simulink model "Regressao9_6"  (R2012b)
settings: Solver=FixedStepDiscrete  SolverMode=SingleTasking  StartTime=0.0  StopTime=limSim  FixedStep=ts  RelTol=1e-3
libraries: xbsIndex_r4 x399, roblocks x1
settings Model: Creator=snata  LastModifiedBy=snata

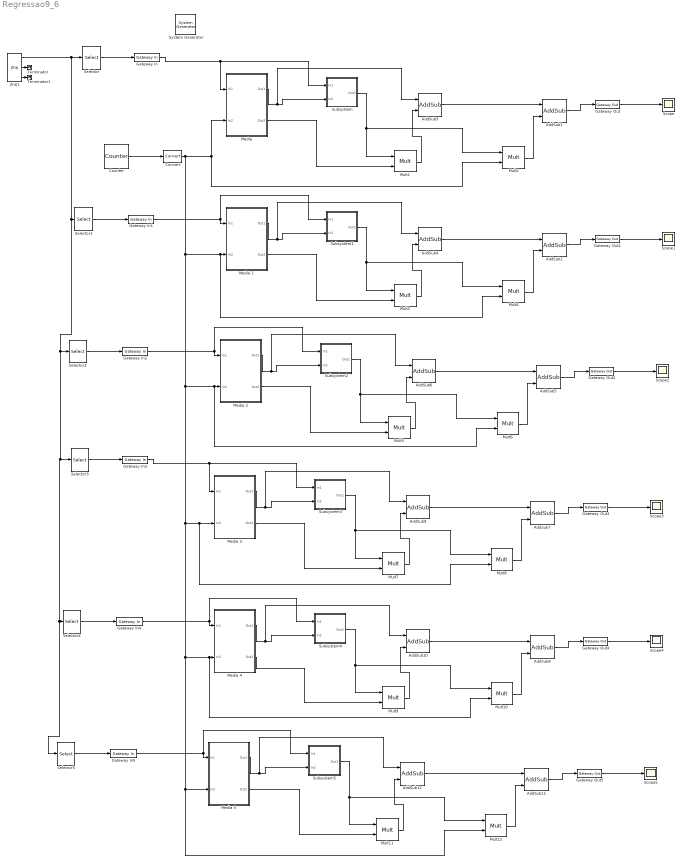
== system Regressao9_6 ==
  " System Generator" : xbsIndex_r4/ System Generator  Tag=genX  xilinxfamily=virtex6  part=xc6vlx240t  speed=-1  package=ff1156  synthesis_tool=XST  clock_wrapper=Clock Enables  directory=C:/Users/snata/Documents/Linear_Predictors/Regressao9/netlist6  proj_type=Project Navigator  Synth_file=XST Defaults  Impl_file=ISE Defaults  testbench=off  simulink_period=ts  sysclk_period=10  dcm_input_clock_period=10  incr_netlist=off  trim_vbits=Everywhere in SubSystem  dbl_ovrd=According to Block Masks  core_generation=According to Block Masks  run_coregen=off  deprecated_control=off  eval_field=0  block_type=sysgen
  AddSub{1..2,5,7..8,11} (6 alike) : xbsIndex_r4/AddSub  mode=Addition  use_carryin=off  use_carryout=off  en=off  latency=0  precision=Full  arith_type=Unsigned  n_bits=16  bin_pt=14  quantization=Truncate  overflow=Wrap  dbl_ovrd=off  use_behavioral_HDL=off  hw_selection=Fabric  pipelined=off  block_type=addsub
  AddSub{3..4,6,9..10,12} (6 alike) : xbsIndex_r4/AddSub  mode=Subtraction  use_carryin=off  use_carryout=off  en=off  latency=0  precision=Full  arith_type=Unsigned  n_bits=16  bin_pt=14  quantization=Truncate  overflow=Wrap  dbl_ovrd=off  use_behavioral_HDL=off  hw_selection=Fabric  pipelined=off  block_type=addsub
  Convert : xbsIndex_r4/Convert  gui_display_data_type=Floating-point  arith_type=Floating-point  n_bits=16  bin_pt=14  float_type=Single  exp_bits=8  fraction_bits=24  quantization=Truncate  overflow=Wrap  en=off  latency=0  dbl_ovrd=off  pipeline=off  block_type=convert
  Counter : xbsIndex_r4/Counter  cnt_type=Free Running  cnt_to=Inf  operation=Up  start_count=0  cnt_by_val=1  arith_type="Signed  (2's comp)"  n_bits=32  bin_pt=1  load_pin=off  rst=off  en=off  explicit_period=on  period=ts  dbl_ovrd=off  use_behavioral_HDL=off  implementation=Fabric  block_type=counter
  Gateway In{,1..5} (6 alike) : xbsIndex_r4/Gateway In  gui_display_data_type=Floating-point  arith_type=Floating-point  n_bits=16  bin_pt=14  preci_type=Single  exp_width=8  frac_width=24  quantization="Round  (unbiased: +/- Inf)"  overflow=Saturate  period=ts  dbl_ovrd=off  timing_constraint=None  locs_specified=off  LOCs={}  UseAsADC=off  ADCChannel='1'  inherit_from_input=off  hdl_port=on  block_type=gatewayin
  Gateway Out{,1..5} (6 alike) : xbsIndex_r4/Gateway Out  inherit_from_input=off  hdl_port=on  timing_constraint=None  locs_specified=off  LOCs={}  UseAsDAC=off  DACChannel='1'  block_type=gatewayout
  "Media " : Subsystem
  Media 1 : Subsystem
  Media 2 : Subsystem
  Media 3 : Subsystem
  Media 4 : Subsystem
  Media 5 : Subsystem
  Mult{1..12} (12 alike) : xbsIndex_r4/Mult  precision=Full  arith_type="Signed  (2's comp)"  n_bits=16  bin_pt=14  quantization=Truncate  overflow=Wrap  en=off  latency=0  dbl_ovrd=off  use_behavioral_HDL=off  opt=Speed  use_embedded=on  optimum_pipeline=off  pipeline=on  use_rpm=on  placement_style=Triangular  block_type=mult
  Scope{,1..5} (6 alike) : Scope
      Scope settings: YMin=5.55112e-17  YMax=1.6
      Scope1 settings: YMin=5.55112e-17  YMax=1.6
      Scope2 settings: YMin=5.55112e-17  YMax=1.6  SaveName=ScopeData2
      Scope3 settings: YMin=5.55112e-17  YMax=1.6  SaveName=ScopeData3
      Scope4 settings: YMin=5.55112e-17  YMax=1.6  SaveName=ScopeData4
      Scope5 settings: YMin=5.55112e-17  YMax=1.6  SaveName=ScopeData5
  Selector{,1..5} (6 alike) : Selector  InputPortWidth=3  IndexOptions=Index vector (dialog)  Indices=[1]  OutputSizes=1
  Subsystem : Subsystem
  Subsystem1 : Subsystem
  Subsystem2 : Subsystem
  Subsystem3 : Subsystem
  Subsystem4 : Subsystem
  Subsystem5 : Subsystem
  Terminator : Terminator
  Terminator1 : Terminator
  jtraj1 : roblocks/Trajectory/jtraj  q0=[0 -pi/2 pi]  qf=[pi/2 pi/4 pi/2]  tmax=limSim  ts=ts
  wires:
  Selector/1 -> Gateway In/1
  Gateway In/1 -> Subsystem/1(In1), "Media "/1(In1)
  AddSub1/1 -> Gateway Out/1
  Gateway Out/1 -> Scope/1
  "Media "/1(Out1) -> AddSub3/1, Subsystem/2(In2)
  Counter/1 -> Convert/1
  Mult1/1 -> AddSub3/2
  AddSub3/1 -> AddSub1/1
  Mult2/1 -> AddSub1/2
  Subsystem/1(Out1) -> Mult2/1, Mult1/1
  "Media "/2(Out2) -> Mult1/2
  Selector1/1 -> Gateway In1/1
  Gateway In1/1 -> Subsystem1/1(In1), Media 1/1(In1)
  AddSub2/1 -> Gateway Out1/1
  Gateway Out1/1 -> Scope1/1
  Media 1/1(Out1) -> AddSub4/1, Subsystem1/2(In2)
  Mult3/1 -> AddSub4/2
  AddSub4/1 -> AddSub2/1
  Mult4/1 -> AddSub2/2
  Subsystem1/1(Out1) -> Mult4/1, Mult3/1
  Media 1/2(Out2) -> Mult3/2
  Selector2/1 -> Gateway In2/1
  Gateway In2/1 -> Subsystem2/1(In1), Media 2/1(In1)
  AddSub5/1 -> Gateway Out2/1
  Gateway Out2/1 -> Scope2/1
  Media 2/1(Out1) -> AddSub6/1, Subsystem2/2(In2)
  Mult5/1 -> AddSub6/2
  AddSub6/1 -> AddSub5/1
  Mult6/1 -> AddSub5/2
  Subsystem2/1(Out1) -> Mult6/1, Mult5/1
  Media 2/2(Out2) -> Mult5/2
  Selector3/1 -> Gateway In3/1
  Gateway In3/1 -> Subsystem3/1(In1), Media 3/1(In1)
  AddSub7/1 -> Gateway Out3/1
  Gateway Out3/1 -> Scope3/1
  Media 3/1(Out1) -> AddSub9/1, Subsystem3/2(In2)
  Mult7/1 -> AddSub9/2
  AddSub9/1 -> AddSub7/1
  Mult8/1 -> AddSub7/2
  Subsystem3/1(Out1) -> Mult8/1, Mult7/1
  Media 3/2(Out2) -> Mult7/2
  Selector4/1 -> Gateway In4/1
  jtraj1/1 -> Selector5/1, Selector4/1, Selector3/1, Selector2/1, Selector1/1, Selector/1
  Gateway In4/1 -> Subsystem4/1(In1), Media 4/1(In1)
  AddSub8/1 -> Gateway Out4/1
  Gateway Out4/1 -> Scope4/1
  Media 4/1(Out1) -> AddSub10/1, Subsystem4/2(In2)
  Mult9/1 -> AddSub10/2
  AddSub10/1 -> AddSub8/1
  Mult10/1 -> AddSub8/2
  Subsystem4/1(Out1) -> Mult10/1, Mult9/1
  Media 4/2(Out2) -> Mult9/2
  Selector5/1 -> Gateway In5/1
  Gateway In5/1 -> Subsystem5/1(In1), Media 5/1(In1)
  AddSub11/1 -> Gateway Out5/1
  Gateway Out5/1 -> Scope5/1
  Media 5/1(Out1) -> AddSub12/1, Subsystem5/2(In2)
  Convert/1 -> Mult4/2, Media 1/2(In2), Mult6/2, Media 2/2(In2), Mult8/2, Media 3/2(In2), Mult10/2, Media 4/2(In2), Media 5/2(In2), Mult12/2, "Media "/2(In2), Mult2/2
  Mult11/1 -> AddSub12/2
  AddSub12/1 -> AddSub11/1
  Mult12/1 -> AddSub11/2
  Subsystem5/1(Out1) -> Mult12/1, Mult11/1
  Media 5/2(Out2) -> Mult11/2
  jtraj1/2 -> Terminator/1
  jtraj1/3 -> Terminator1/1

== system Regressao9_6/Media  ==
  In1 : Inport
  In2 : Inport  Port=2
  CMult : xbsIndex_r4/CMult  const=1/10  gui_display_data_type=Floating-point  const_n_bits=16  const_bin_pt=14  float_type=Single  exp_bits=8  fraction_bits=24  en=off  latency=0  precision=Full  arith_type="Signed  (2's comp)"  n_bits=16  bin_pt=14  quantization=Truncate  overflow=Wrap  dbl_ovrd=off  use_behavioral_HDL=off  mem_type=Distributed RAM  pipeline=off  block_type=cmult
  CMult1 : xbsIndex_r4/CMult  const=1/10  gui_display_data_type=Floating-point  const_n_bits=16  const_bin_pt=14  float_type=Single  exp_bits=8  fraction_bits=24  en=off  latency=0  precision=Full  arith_type="Signed  (2's comp)"  n_bits=16  bin_pt=14  quantization=Truncate  overflow=Wrap  dbl_ovrd=off  use_behavioral_HDL=off  mem_type=Distributed RAM  pipeline=off  block_type=cmult
  Soma : Subsystem
  Soma1 : Subsystem
  Out1 : Outport
  Out2 : Outport  Port=2
  wires:
  In1/1 -> Soma/1(In1)
  Soma/1(Out1) -> CMult/1
  CMult/1 -> Out1/1
  In2/1 -> Soma1/1(In1)
  Soma1/1(Out1) -> CMult1/1
  CMult1/1 -> Out2/1

== system Regressao9_6/Media 1 ==
  In1 : Inport
  In2 : Inport  Port=2
  CMult : xbsIndex_r4/CMult  const=1/10  gui_display_data_type=Floating-point  const_n_bits=16  const_bin_pt=14  float_type=Single  exp_bits=8  fraction_bits=24  en=off  latency=0  precision=Full  arith_type="Signed  (2's comp)"  n_bits=16  bin_pt=14  quantization=Truncate  overflow=Wrap  dbl_ovrd=off  use_behavioral_HDL=off  mem_type=Distributed RAM  pipeline=off  block_type=cmult
  CMult1 : xbsIndex_r4/CMult  const=1/10  gui_display_data_type=Floating-point  const_n_bits=16  const_bin_pt=14  float_type=Single  exp_bits=8  fraction_bits=24  en=off  latency=0  precision=Full  arith_type="Signed  (2's comp)"  n_bits=16  bin_pt=14  quantization=Truncate  overflow=Wrap  dbl_ovrd=off  use_behavioral_HDL=off  mem_type=Distributed RAM  pipeline=off  block_type=cmult
  Soma : Subsystem
  Soma1 : Subsystem
  Out1 : Outport
  Out2 : Outport  Port=2
  wires:
  In1/1 -> Soma/1(In1)
  Soma/1(Out1) -> CMult/1
  CMult/1 -> Out1/1
  In2/1 -> Soma1/1(In1)
  Soma1/1(Out1) -> CMult1/1
  CMult1/1 -> Out2/1

== system Regressao9_6/Media 2 ==
  In1 : Inport
  In2 : Inport  Port=2
  CMult : xbsIndex_r4/CMult  const=1/10  gui_display_data_type=Floating-point  const_n_bits=16  const_bin_pt=14  float_type=Single  exp_bits=8  fraction_bits=24  en=off  latency=0  precision=Full  arith_type="Signed  (2's comp)"  n_bits=16  bin_pt=14  quantization=Truncate  overflow=Wrap  dbl_ovrd=off  use_behavioral_HDL=off  mem_type=Distributed RAM  pipeline=off  block_type=cmult
  CMult1 : xbsIndex_r4/CMult  const=1/10  gui_display_data_type=Floating-point  const_n_bits=16  const_bin_pt=14  float_type=Single  exp_bits=8  fraction_bits=24  en=off  latency=0  precision=Full  arith_type="Signed  (2's comp)"  n_bits=16  bin_pt=14  quantization=Truncate  overflow=Wrap  dbl_ovrd=off  use_behavioral_HDL=off  mem_type=Distributed RAM  pipeline=off  block_type=cmult
  Soma : Subsystem
  Soma1 : Subsystem
  Out1 : Outport
  Out2 : Outport  Port=2
  wires:
  In1/1 -> Soma/1(In1)
  Soma/1(Out1) -> CMult/1
  CMult/1 -> Out1/1
  In2/1 -> Soma1/1(In1)
  Soma1/1(Out1) -> CMult1/1
  CMult1/1 -> Out2/1

== system Regressao9_6/Media 3 ==
  In1 : Inport
  In2 : Inport  Port=2
  CMult : xbsIndex_r4/CMult  const=1/10  gui_display_data_type=Floating-point  const_n_bits=16  const_bin_pt=14  float_type=Single  exp_bits=8  fraction_bits=24  en=off  latency=0  precision=Full  arith_type="Signed  (2's comp)"  n_bits=16  bin_pt=14  quantization=Truncate  overflow=Wrap  dbl_ovrd=off  use_behavioral_HDL=off  mem_type=Distributed RAM  pipeline=off  block_type=cmult
  CMult1 : xbsIndex_r4/CMult  const=1/10  gui_display_data_type=Floating-point  const_n_bits=16  const_bin_pt=14  float_type=Single  exp_bits=8  fraction_bits=24  en=off  latency=0  precision=Full  arith_type="Signed  (2's comp)"  n_bits=16  bin_pt=14  quantization=Truncate  overflow=Wrap  dbl_ovrd=off  use_behavioral_HDL=off  mem_type=Distributed RAM  pipeline=off  block_type=cmult
  Soma : Subsystem
  Soma1 : Subsystem
  Out1 : Outport
  Out2 : Outport  Port=2
  wires:
  In1/1 -> Soma/1(In1)
  Soma/1(Out1) -> CMult/1
  CMult/1 -> Out1/1
  In2/1 -> Soma1/1(In1)
  Soma1/1(Out1) -> CMult1/1
  CMult1/1 -> Out2/1

== system Regressao9_6/Media 4 ==
  In1 : Inport
  In2 : Inport  Port=2
  CMult : xbsIndex_r4/CMult  const=1/10  gui_display_data_type=Floating-point  const_n_bits=16  const_bin_pt=14  float_type=Single  exp_bits=8  fraction_bits=24  en=off  latency=0  precision=Full  arith_type="Signed  (2's comp)"  n_bits=16  bin_pt=14  quantization=Truncate  overflow=Wrap  dbl_ovrd=off  use_behavioral_HDL=off  mem_type=Distributed RAM  pipeline=off  block_type=cmult
  CMult1 : xbsIndex_r4/CMult  const=1/10  gui_display_data_type=Floating-point  const_n_bits=16  const_bin_pt=14  float_type=Single  exp_bits=8  fraction_bits=24  en=off  latency=0  precision=Full  arith_type="Signed  (2's comp)"  n_bits=16  bin_pt=14  quantization=Truncate  overflow=Wrap  dbl_ovrd=off  use_behavioral_HDL=off  mem_type=Distributed RAM  pipeline=off  block_type=cmult
  Soma : Subsystem
  Soma1 : Subsystem
  Out1 : Outport
  Out2 : Outport  Port=2
  wires:
  In1/1 -> Soma/1(In1)
  Soma/1(Out1) -> CMult/1
  CMult/1 -> Out1/1
  In2/1 -> Soma1/1(In1)
  Soma1/1(Out1) -> CMult1/1
  CMult1/1 -> Out2/1

== system Regressao9_6/Media 5 ==
  In1 : Inport
  In2 : Inport  Port=2
  CMult : xbsIndex_r4/CMult  const=1/10  gui_display_data_type=Floating-point  const_n_bits=16  const_bin_pt=14  float_type=Single  exp_bits=8  fraction_bits=24  en=off  latency=0  precision=Full  arith_type="Signed  (2's comp)"  n_bits=16  bin_pt=14  quantization=Truncate  overflow=Wrap  dbl_ovrd=off  use_behavioral_HDL=off  mem_type=Distributed RAM  pipeline=off  block_type=cmult
  CMult1 : xbsIndex_r4/CMult  const=1/10  gui_display_data_type=Floating-point  const_n_bits=16  const_bin_pt=14  float_type=Single  exp_bits=8  fraction_bits=24  en=off  latency=0  precision=Full  arith_type="Signed  (2's comp)"  n_bits=16  bin_pt=14  quantization=Truncate  overflow=Wrap  dbl_ovrd=off  use_behavioral_HDL=off  mem_type=Distributed RAM  pipeline=off  block_type=cmult
  Soma : Subsystem
  Soma1 : Subsystem
  Out1 : Outport
  Out2 : Outport  Port=2
  wires:
  In1/1 -> Soma/1(In1)
  Soma/1(Out1) -> CMult/1
  CMult/1 -> Out1/1
  In2/1 -> Soma1/1(In1)
  Soma1/1(Out1) -> CMult1/1
  CMult1/1 -> Out2/1

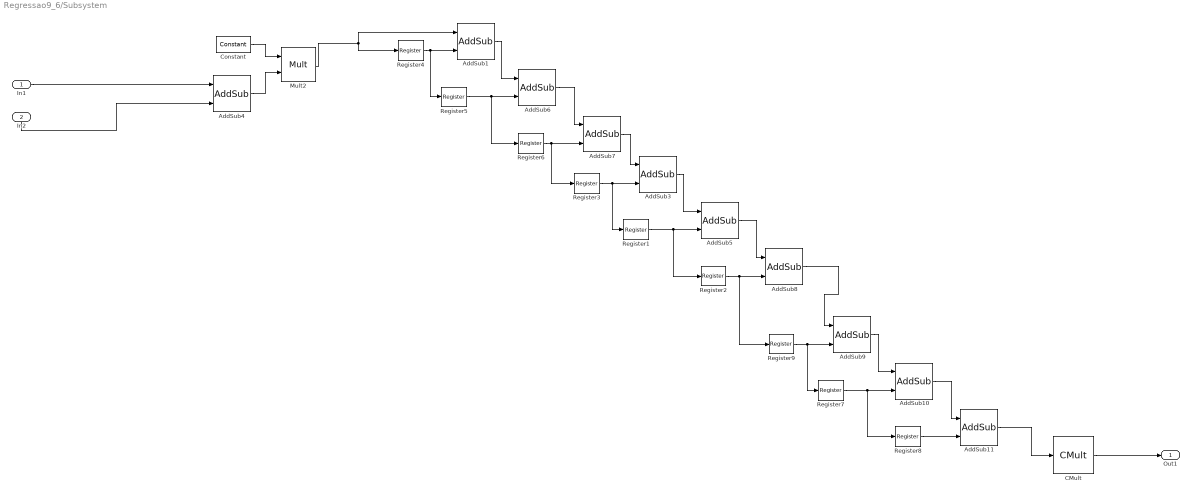
== system Regressao9_6/Subsystem ==
  In1 : Inport
  In2 : Inport  Port=2
  AddSub{1,3,5..11} (9 alike) : xbsIndex_r4/AddSub  mode=Addition  use_carryin=off  use_carryout=off  en=off  latency=0  precision=Full  arith_type=Unsigned  n_bits=16  bin_pt=14  quantization=Truncate  overflow=Wrap  dbl_ovrd=off  use_behavioral_HDL=off  hw_selection=Fabric  pipelined=off  block_type=addsub
  AddSub4 : xbsIndex_r4/AddSub  mode=Subtraction  use_carryin=off  use_carryout=off  en=off  latency=0  precision=Full  arith_type=Unsigned  n_bits=16  bin_pt=14  quantization=Truncate  overflow=Wrap  dbl_ovrd=off  use_behavioral_HDL=off  hw_selection=Fabric  pipelined=off  block_type=addsub
  CMult : xbsIndex_r4/CMult  const=1/20.25  gui_display_data_type=Floating-point  const_n_bits=16  const_bin_pt=14  float_type=Single  exp_bits=8  fraction_bits=24  en=off  latency=0  precision=Full  arith_type="Signed  (2's comp)"  n_bits=16  bin_pt=14  quantization=Truncate  overflow=Wrap  dbl_ovrd=off  use_behavioral_HDL=off  mem_type=Distributed RAM  pipeline=off  block_type=cmult
  Constant : xbsIndex_r4/Constant  const=4.5  gui_display_data_type=Floating-point  arith_type=Floating-point  n_bits=16  bin_pt=14  preci_type=Single  exp_width=8  frac_width=24  explicit_period=off  period=1  equ=P=C  opselect=C  inp2=PCIN>>17  opr=+  inp1=P  carry=CIN  dbl_ovrd=off  block_type=constant
  Mult2 : xbsIndex_r4/Mult  precision=Full  arith_type="Signed  (2's comp)"  n_bits=16  bin_pt=14  quantization=Truncate  overflow=Wrap  en=off  latency=0  dbl_ovrd=off  use_behavioral_HDL=off  opt=Speed  use_embedded=on  optimum_pipeline=off  pipeline=on  use_rpm=on  placement_style=Triangular  block_type=mult
  Register{1..9} (9 alike) : xbsIndex_r4/Register  init=0  rst=off  en=off  dbl_ovrd=off  block_type=register
  Out1 : Outport
  wires:
  CMult/1 -> Out1/1
  AddSub4/1 -> Mult2/2
  In1/1 -> AddSub4/1
  In2/1 -> AddSub4/2
  AddSub11/1 -> CMult/1
  Mult2/1 -> Register4/1, AddSub1/1
  AddSub6/1 -> AddSub7/1
  AddSub1/1 -> AddSub6/1
  Register4/1 -> Register5/1, AddSub1/2
  Register5/1 -> Register6/1, AddSub6/2
  Register6/1 -> Register3/1, AddSub7/2
  AddSub5/1 -> AddSub8/1
  AddSub3/1 -> AddSub5/1
  Register3/1 -> Register1/1, AddSub3/2
  Register1/1 -> Register2/1, AddSub5/2
  AddSub7/1 -> AddSub3/1
  Register2/1 -> Register9/1, AddSub8/2
  AddSub10/1 -> AddSub11/1
  AddSub9/1 -> AddSub10/1
  Register9/1 -> AddSub9/2, Register7/1
  Register7/1 -> AddSub10/2, Register8/1
  Register8/1 -> AddSub11/2
  AddSub8/1 -> AddSub9/1
  Constant/1 -> Mult2/1

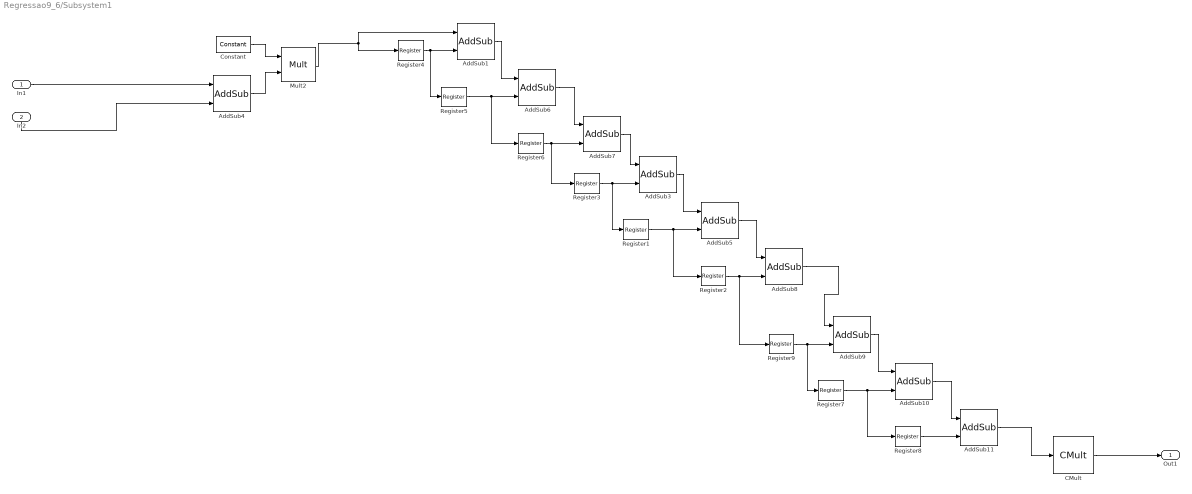
== system Regressao9_6/Subsystem1 ==
  In1 : Inport
  In2 : Inport  Port=2
  AddSub{1,3,5..11} (9 alike) : xbsIndex_r4/AddSub  mode=Addition  use_carryin=off  use_carryout=off  en=off  latency=0  precision=Full  arith_type=Unsigned  n_bits=16  bin_pt=14  quantization=Truncate  overflow=Wrap  dbl_ovrd=off  use_behavioral_HDL=off  hw_selection=Fabric  pipelined=off  block_type=addsub
  AddSub4 : xbsIndex_r4/AddSub  mode=Subtraction  use_carryin=off  use_carryout=off  en=off  latency=0  precision=Full  arith_type=Unsigned  n_bits=16  bin_pt=14  quantization=Truncate  overflow=Wrap  dbl_ovrd=off  use_behavioral_HDL=off  hw_selection=Fabric  pipelined=off  block_type=addsub
  CMult : xbsIndex_r4/CMult  const=1/20.25  gui_display_data_type=Floating-point  const_n_bits=16  const_bin_pt=14  float_type=Single  exp_bits=8  fraction_bits=24  en=off  latency=0  precision=Full  arith_type="Signed  (2's comp)"  n_bits=16  bin_pt=14  quantization=Truncate  overflow=Wrap  dbl_ovrd=off  use_behavioral_HDL=off  mem_type=Distributed RAM  pipeline=off  block_type=cmult
  Constant : xbsIndex_r4/Constant  const=4.5  gui_display_data_type=Floating-point  arith_type=Floating-point  n_bits=16  bin_pt=14  preci_type=Single  exp_width=8  frac_width=24  explicit_period=off  period=1  equ=P=C  opselect=C  inp2=PCIN>>17  opr=+  inp1=P  carry=CIN  dbl_ovrd=off  block_type=constant
  Mult2 : xbsIndex_r4/Mult  precision=Full  arith_type="Signed  (2's comp)"  n_bits=16  bin_pt=14  quantization=Truncate  overflow=Wrap  en=off  latency=0  dbl_ovrd=off  use_behavioral_HDL=off  opt=Speed  use_embedded=on  optimum_pipeline=off  pipeline=on  use_rpm=on  placement_style=Triangular  block_type=mult
  Register{1..9} (9 alike) : xbsIndex_r4/Register  init=0  rst=off  en=off  dbl_ovrd=off  block_type=register
  Out1 : Outport
  wires:
  CMult/1 -> Out1/1
  AddSub4/1 -> Mult2/2
  In1/1 -> AddSub4/1
  In2/1 -> AddSub4/2
  AddSub11/1 -> CMult/1
  Mult2/1 -> Register4/1, AddSub1/1
  AddSub6/1 -> AddSub7/1
  AddSub1/1 -> AddSub6/1
  Register4/1 -> Register5/1, AddSub1/2
  Register5/1 -> Register6/1, AddSub6/2
  Register6/1 -> Register3/1, AddSub7/2
  AddSub5/1 -> AddSub8/1
  AddSub3/1 -> AddSub5/1
  Register3/1 -> Register1/1, AddSub3/2
  Register1/1 -> Register2/1, AddSub5/2
  AddSub7/1 -> AddSub3/1
  Register2/1 -> Register9/1, AddSub8/2
  AddSub10/1 -> AddSub11/1
  AddSub9/1 -> AddSub10/1
  Register9/1 -> AddSub9/2, Register7/1
  Register7/1 -> AddSub10/2, Register8/1
  Register8/1 -> AddSub11/2
  AddSub8/1 -> AddSub9/1
  Constant/1 -> Mult2/1

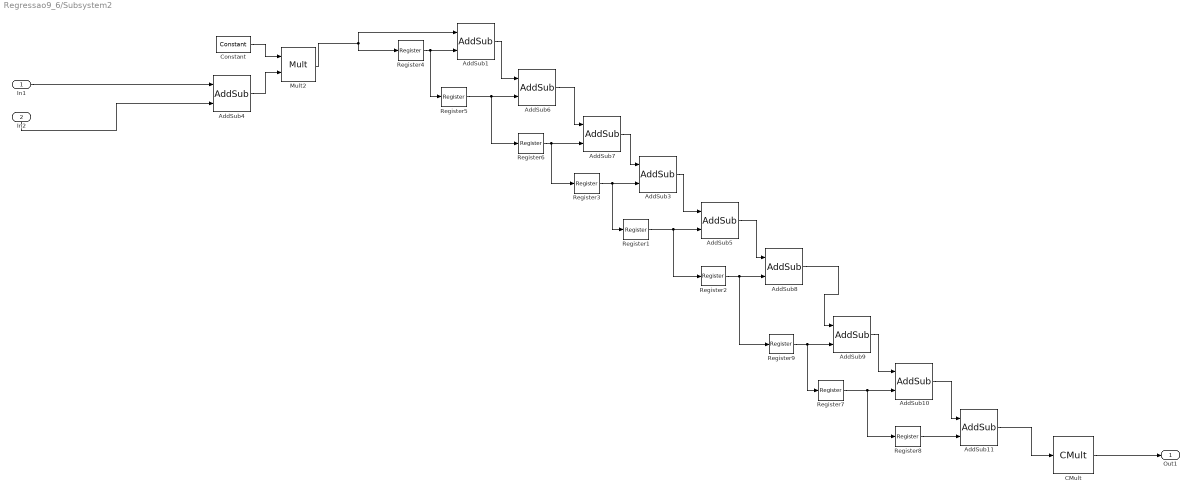
== system Regressao9_6/Subsystem2 ==
  In1 : Inport
  In2 : Inport  Port=2
  AddSub{1,3,5..11} (9 alike) : xbsIndex_r4/AddSub  mode=Addition  use_carryin=off  use_carryout=off  en=off  latency=0  precision=Full  arith_type=Unsigned  n_bits=16  bin_pt=14  quantization=Truncate  overflow=Wrap  dbl_ovrd=off  use_behavioral_HDL=off  hw_selection=Fabric  pipelined=off  block_type=addsub
  AddSub4 : xbsIndex_r4/AddSub  mode=Subtraction  use_carryin=off  use_carryout=off  en=off  latency=0  precision=Full  arith_type=Unsigned  n_bits=16  bin_pt=14  quantization=Truncate  overflow=Wrap  dbl_ovrd=off  use_behavioral_HDL=off  hw_selection=Fabric  pipelined=off  block_type=addsub
  CMult : xbsIndex_r4/CMult  const=1/20.25  gui_display_data_type=Floating-point  const_n_bits=16  const_bin_pt=14  float_type=Single  exp_bits=8  fraction_bits=24  en=off  latency=0  precision=Full  arith_type="Signed  (2's comp)"  n_bits=16  bin_pt=14  quantization=Truncate  overflow=Wrap  dbl_ovrd=off  use_behavioral_HDL=off  mem_type=Distributed RAM  pipeline=off  block_type=cmult
  Constant : xbsIndex_r4/Constant  const=4.5  gui_display_data_type=Floating-point  arith_type=Floating-point  n_bits=16  bin_pt=14  preci_type=Single  exp_width=8  frac_width=24  explicit_period=off  period=1  equ=P=C  opselect=C  inp2=PCIN>>17  opr=+  inp1=P  carry=CIN  dbl_ovrd=off  block_type=constant
  Mult2 : xbsIndex_r4/Mult  precision=Full  arith_type="Signed  (2's comp)"  n_bits=16  bin_pt=14  quantization=Truncate  overflow=Wrap  en=off  latency=0  dbl_ovrd=off  use_behavioral_HDL=off  opt=Speed  use_embedded=on  optimum_pipeline=off  pipeline=on  use_rpm=on  placement_style=Triangular  block_type=mult
  Register{1..9} (9 alike) : xbsIndex_r4/Register  init=0  rst=off  en=off  dbl_ovrd=off  block_type=register
  Out1 : Outport
  wires:
  CMult/1 -> Out1/1
  AddSub4/1 -> Mult2/2
  In1/1 -> AddSub4/1
  In2/1 -> AddSub4/2
  AddSub11/1 -> CMult/1
  Mult2/1 -> Register4/1, AddSub1/1
  AddSub6/1 -> AddSub7/1
  AddSub1/1 -> AddSub6/1
  Register4/1 -> Register5/1, AddSub1/2
  Register5/1 -> Register6/1, AddSub6/2
  Register6/1 -> Register3/1, AddSub7/2
  AddSub5/1 -> AddSub8/1
  AddSub3/1 -> AddSub5/1
  Register3/1 -> Register1/1, AddSub3/2
  Register1/1 -> Register2/1, AddSub5/2
  AddSub7/1 -> AddSub3/1
  Register2/1 -> Register9/1, AddSub8/2
  AddSub10/1 -> AddSub11/1
  AddSub9/1 -> AddSub10/1
  Register9/1 -> AddSub9/2, Register7/1
  Register7/1 -> AddSub10/2, Register8/1
  Register8/1 -> AddSub11/2
  AddSub8/1 -> AddSub9/1
  Constant/1 -> Mult2/1

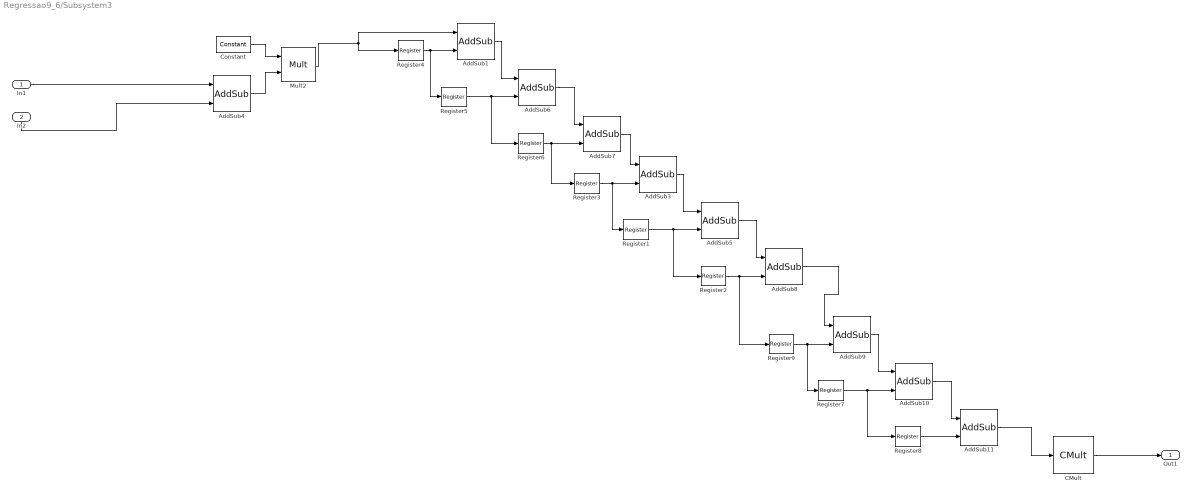
== system Regressao9_6/Subsystem3 ==
  In1 : Inport
  In2 : Inport  Port=2
  AddSub{1,3,5..11} (9 alike) : xbsIndex_r4/AddSub  mode=Addition  use_carryin=off  use_carryout=off  en=off  latency=0  precision=Full  arith_type=Unsigned  n_bits=16  bin_pt=14  quantization=Truncate  overflow=Wrap  dbl_ovrd=off  use_behavioral_HDL=off  hw_selection=Fabric  pipelined=off  block_type=addsub
  AddSub4 : xbsIndex_r4/AddSub  mode=Subtraction  use_carryin=off  use_carryout=off  en=off  latency=0  precision=Full  arith_type=Unsigned  n_bits=16  bin_pt=14  quantization=Truncate  overflow=Wrap  dbl_ovrd=off  use_behavioral_HDL=off  hw_selection=Fabric  pipelined=off  block_type=addsub
  CMult : xbsIndex_r4/CMult  const=1/20.25  gui_display_data_type=Floating-point  const_n_bits=16  const_bin_pt=14  float_type=Single  exp_bits=8  fraction_bits=24  en=off  latency=0  precision=Full  arith_type="Signed  (2's comp)"  n_bits=16  bin_pt=14  quantization=Truncate  overflow=Wrap  dbl_ovrd=off  use_behavioral_HDL=off  mem_type=Distributed RAM  pipeline=off  block_type=cmult
  Constant : xbsIndex_r4/Constant  const=4.5  gui_display_data_type=Floating-point  arith_type=Floating-point  n_bits=16  bin_pt=14  preci_type=Single  exp_width=8  frac_width=24  explicit_period=off  period=1  equ=P=C  opselect=C  inp2=PCIN>>17  opr=+  inp1=P  carry=CIN  dbl_ovrd=off  block_type=constant
  Mult2 : xbsIndex_r4/Mult  precision=Full  arith_type="Signed  (2's comp)"  n_bits=16  bin_pt=14  quantization=Truncate  overflow=Wrap  en=off  latency=0  dbl_ovrd=off  use_behavioral_HDL=off  opt=Speed  use_embedded=on  optimum_pipeline=off  pipeline=on  use_rpm=on  placement_style=Triangular  block_type=mult
  Register{1..9} (9 alike) : xbsIndex_r4/Register  init=0  rst=off  en=off  dbl_ovrd=off  block_type=register
  Out1 : Outport
  wires:
  CMult/1 -> Out1/1
  AddSub4/1 -> Mult2/2
  In1/1 -> AddSub4/1
  In2/1 -> AddSub4/2
  AddSub11/1 -> CMult/1
  Mult2/1 -> Register4/1, AddSub1/1
  AddSub6/1 -> AddSub7/1
  AddSub1/1 -> AddSub6/1
  Register4/1 -> Register5/1, AddSub1/2
  Register5/1 -> Register6/1, AddSub6/2
  Register6/1 -> Register3/1, AddSub7/2
  AddSub5/1 -> AddSub8/1
  AddSub3/1 -> AddSub5/1
  Register3/1 -> Register1/1, AddSub3/2
  Register1/1 -> Register2/1, AddSub5/2
  AddSub7/1 -> AddSub3/1
  Register2/1 -> Register9/1, AddSub8/2
  AddSub10/1 -> AddSub11/1
  AddSub9/1 -> AddSub10/1
  Register9/1 -> AddSub9/2, Register7/1
  Register7/1 -> AddSub10/2, Register8/1
  Register8/1 -> AddSub11/2
  AddSub8/1 -> AddSub9/1
  Constant/1 -> Mult2/1

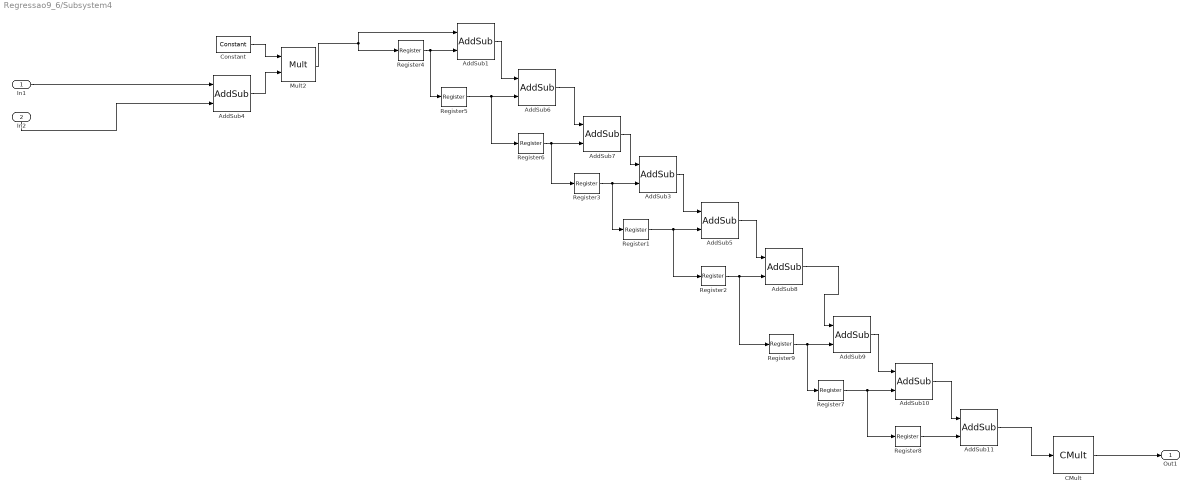
== system Regressao9_6/Subsystem4 ==
  In1 : Inport
  In2 : Inport  Port=2
  AddSub{1,3,5..11} (9 alike) : xbsIndex_r4/AddSub  mode=Addition  use_carryin=off  use_carryout=off  en=off  latency=0  precision=Full  arith_type=Unsigned  n_bits=16  bin_pt=14  quantization=Truncate  overflow=Wrap  dbl_ovrd=off  use_behavioral_HDL=off  hw_selection=Fabric  pipelined=off  block_type=addsub
  AddSub4 : xbsIndex_r4/AddSub  mode=Subtraction  use_carryin=off  use_carryout=off  en=off  latency=0  precision=Full  arith_type=Unsigned  n_bits=16  bin_pt=14  quantization=Truncate  overflow=Wrap  dbl_ovrd=off  use_behavioral_HDL=off  hw_selection=Fabric  pipelined=off  block_type=addsub
  CMult : xbsIndex_r4/CMult  const=1/20.25  gui_display_data_type=Floating-point  const_n_bits=16  const_bin_pt=14  float_type=Single  exp_bits=8  fraction_bits=24  en=off  latency=0  precision=Full  arith_type="Signed  (2's comp)"  n_bits=16  bin_pt=14  quantization=Truncate  overflow=Wrap  dbl_ovrd=off  use_behavioral_HDL=off  mem_type=Distributed RAM  pipeline=off  block_type=cmult
  Constant : xbsIndex_r4/Constant  const=4.5  gui_display_data_type=Floating-point  arith_type=Floating-point  n_bits=16  bin_pt=14  preci_type=Single  exp_width=8  frac_width=24  explicit_period=off  period=1  equ=P=C  opselect=C  inp2=PCIN>>17  opr=+  inp1=P  carry=CIN  dbl_ovrd=off  block_type=constant
  Mult2 : xbsIndex_r4/Mult  precision=Full  arith_type="Signed  (2's comp)"  n_bits=16  bin_pt=14  quantization=Truncate  overflow=Wrap  en=off  latency=0  dbl_ovrd=off  use_behavioral_HDL=off  opt=Speed  use_embedded=on  optimum_pipeline=off  pipeline=on  use_rpm=on  placement_style=Triangular  block_type=mult
  Register{1..9} (9 alike) : xbsIndex_r4/Register  init=0  rst=off  en=off  dbl_ovrd=off  block_type=register
  Out1 : Outport
  wires:
  CMult/1 -> Out1/1
  AddSub4/1 -> Mult2/2
  In1/1 -> AddSub4/1
  In2/1 -> AddSub4/2
  AddSub11/1 -> CMult/1
  Mult2/1 -> Register4/1, AddSub1/1
  AddSub6/1 -> AddSub7/1
  AddSub1/1 -> AddSub6/1
  Register4/1 -> Register5/1, AddSub1/2
  Register5/1 -> Register6/1, AddSub6/2
  Register6/1 -> Register3/1, AddSub7/2
  AddSub5/1 -> AddSub8/1
  AddSub3/1 -> AddSub5/1
  Register3/1 -> Register1/1, AddSub3/2
  Register1/1 -> Register2/1, AddSub5/2
  AddSub7/1 -> AddSub3/1
  Register2/1 -> Register9/1, AddSub8/2
  AddSub10/1 -> AddSub11/1
  AddSub9/1 -> AddSub10/1
  Register9/1 -> AddSub9/2, Register7/1
  Register7/1 -> AddSub10/2, Register8/1
  Register8/1 -> AddSub11/2
  AddSub8/1 -> AddSub9/1
  Constant/1 -> Mult2/1

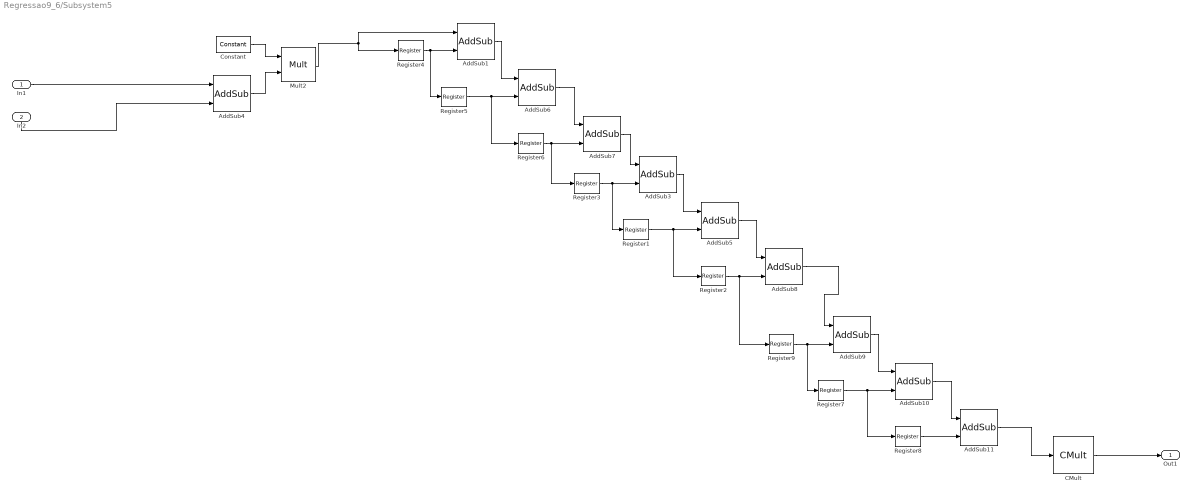
== system Regressao9_6/Subsystem5 ==
  In1 : Inport
  In2 : Inport  Port=2
  AddSub{1,3,5..11} (9 alike) : xbsIndex_r4/AddSub  mode=Addition  use_carryin=off  use_carryout=off  en=off  latency=0  precision=Full  arith_type=Unsigned  n_bits=16  bin_pt=14  quantization=Truncate  overflow=Wrap  dbl_ovrd=off  use_behavioral_HDL=off  hw_selection=Fabric  pipelined=off  block_type=addsub
  AddSub4 : xbsIndex_r4/AddSub  mode=Subtraction  use_carryin=off  use_carryout=off  en=off  latency=0  precision=Full  arith_type=Unsigned  n_bits=16  bin_pt=14  quantization=Truncate  overflow=Wrap  dbl_ovrd=off  use_behavioral_HDL=off  hw_selection=Fabric  pipelined=off  block_type=addsub
  CMult : xbsIndex_r4/CMult  const=1/20.25  gui_display_data_type=Floating-point  const_n_bits=16  const_bin_pt=14  float_type=Single  exp_bits=8  fraction_bits=24  en=off  latency=0  precision=Full  arith_type="Signed  (2's comp)"  n_bits=16  bin_pt=14  quantization=Truncate  overflow=Wrap  dbl_ovrd=off  use_behavioral_HDL=off  mem_type=Distributed RAM  pipeline=off  block_type=cmult
  Constant : xbsIndex_r4/Constant  const=4.5  gui_display_data_type=Floating-point  arith_type=Floating-point  n_bits=16  bin_pt=14  preci_type=Single  exp_width=8  frac_width=24  explicit_period=off  period=1  equ=P=C  opselect=C  inp2=PCIN>>17  opr=+  inp1=P  carry=CIN  dbl_ovrd=off  block_type=constant
  Mult2 : xbsIndex_r4/Mult  precision=Full  arith_type="Signed  (2's comp)"  n_bits=16  bin_pt=14  quantization=Truncate  overflow=Wrap  en=off  latency=0  dbl_ovrd=off  use_behavioral_HDL=off  opt=Speed  use_embedded=on  optimum_pipeline=off  pipeline=on  use_rpm=on  placement_style=Triangular  block_type=mult
  Register{1..9} (9 alike) : xbsIndex_r4/Register  init=0  rst=off  en=off  dbl_ovrd=off  block_type=register
  Out1 : Outport
  wires:
  CMult/1 -> Out1/1
  AddSub4/1 -> Mult2/2
  In1/1 -> AddSub4/1
  In2/1 -> AddSub4/2
  AddSub11/1 -> CMult/1
  Mult2/1 -> Register4/1, AddSub1/1
  AddSub6/1 -> AddSub7/1
  AddSub1/1 -> AddSub6/1
  Register4/1 -> Register5/1, AddSub1/2
  Register5/1 -> Register6/1, AddSub6/2
  Register6/1 -> Register3/1, AddSub7/2
  AddSub5/1 -> AddSub8/1
  AddSub3/1 -> AddSub5/1
  Register3/1 -> Register1/1, AddSub3/2
  Register1/1 -> Register2/1, AddSub5/2
  AddSub7/1 -> AddSub3/1
  Register2/1 -> Register9/1, AddSub8/2
  AddSub10/1 -> AddSub11/1
  AddSub9/1 -> AddSub10/1
  Register9/1 -> AddSub9/2, Register7/1
  Register7/1 -> AddSub10/2, Register8/1
  Register8/1 -> AddSub11/2
  AddSub8/1 -> AddSub9/1
  Constant/1 -> Mult2/1

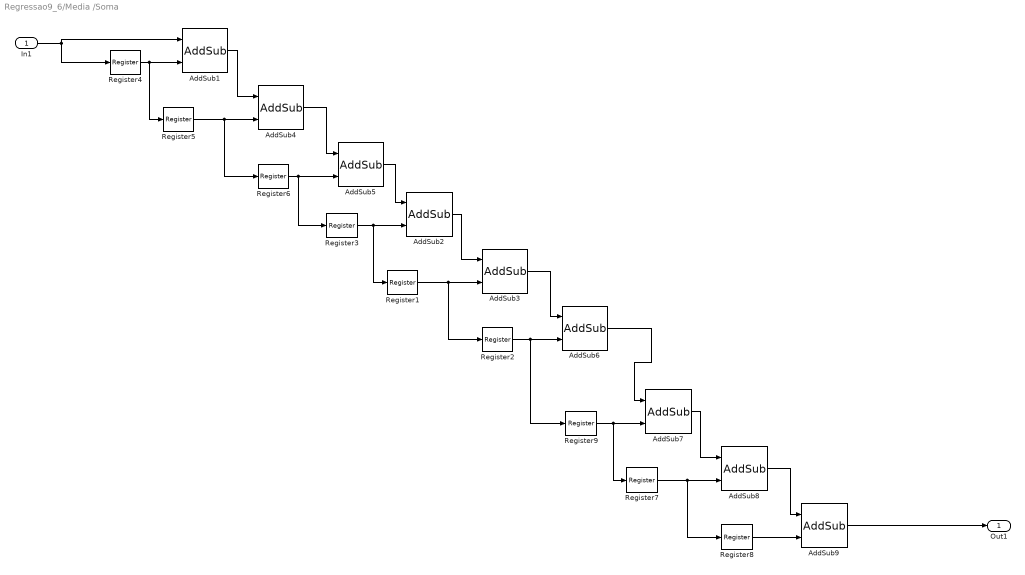
== system Regressao9_6/Media /Soma ==
  In1 : Inport
  AddSub{1..9} (9 alike) : xbsIndex_r4/AddSub  mode=Addition  use_carryin=off  use_carryout=off  en=off  latency=0  precision=Full  arith_type=Unsigned  n_bits=16  bin_pt=14  quantization=Truncate  overflow=Wrap  dbl_ovrd=off  use_behavioral_HDL=off  hw_selection=Fabric  pipelined=off  block_type=addsub
  Register{1..9} (9 alike) : xbsIndex_r4/Register  init=0  rst=off  en=off  dbl_ovrd=off  block_type=register
  Out1 : Outport
  wires:
  AddSub9/1 -> Out1/1
  In1/1 -> AddSub1/1, Register4/1
  AddSub4/1 -> AddSub5/1
  AddSub1/1 -> AddSub4/1
  Register4/1 -> Register5/1, AddSub1/2
  Register5/1 -> Register6/1, AddSub4/2
  Register6/1 -> Register3/1, AddSub5/2
  AddSub3/1 -> AddSub6/1
  AddSub2/1 -> AddSub3/1
  Register3/1 -> Register1/1, AddSub2/2
  Register1/1 -> Register2/1, AddSub3/2
  AddSub5/1 -> AddSub2/1
  Register2/1 -> Register9/1, AddSub6/2
  AddSub8/1 -> AddSub9/1
  AddSub7/1 -> AddSub8/1
  Register9/1 -> AddSub7/2, Register7/1
  Register7/1 -> AddSub8/2, Register8/1
  Register8/1 -> AddSub9/2
  AddSub6/1 -> AddSub7/1

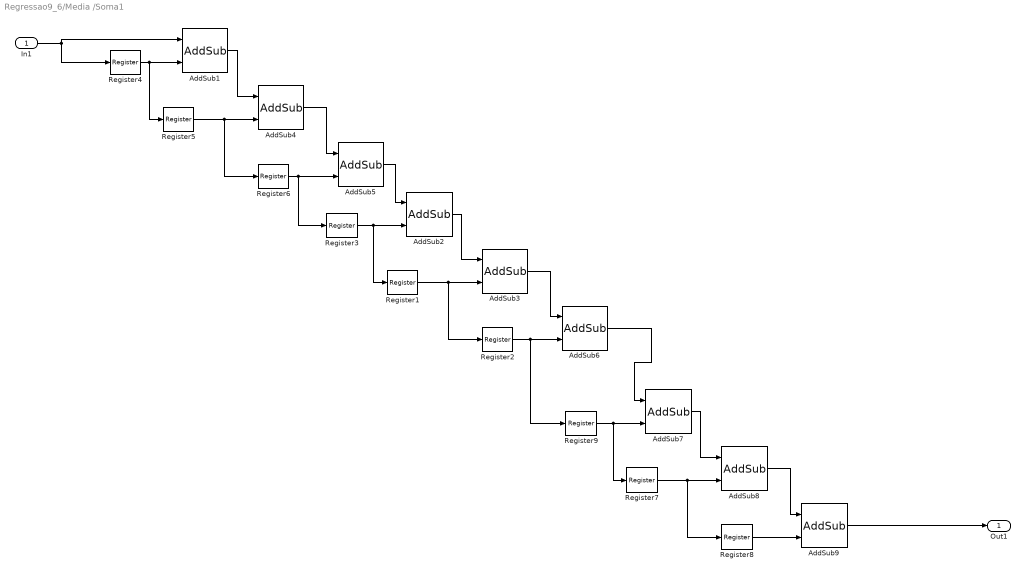
== system Regressao9_6/Media /Soma1 ==
  In1 : Inport
  AddSub{1..9} (9 alike) : xbsIndex_r4/AddSub  mode=Addition  use_carryin=off  use_carryout=off  en=off  latency=0  precision=Full  arith_type=Unsigned  n_bits=16  bin_pt=14  quantization=Truncate  overflow=Wrap  dbl_ovrd=off  use_behavioral_HDL=off  hw_selection=Fabric  pipelined=off  block_type=addsub
  Register{1..9} (9 alike) : xbsIndex_r4/Register  init=0  rst=off  en=off  dbl_ovrd=off  block_type=register
  Out1 : Outport
  wires:
  AddSub6/1 -> AddSub7/1
  Register8/1 -> AddSub9/2
  Register7/1 -> Register8/1, AddSub8/2
  Register9/1 -> Register7/1, AddSub7/2
  AddSub7/1 -> AddSub8/1
  AddSub8/1 -> AddSub9/1
  Register2/1 -> AddSub6/2, Register9/1
  AddSub5/1 -> AddSub2/1
  Register1/1 -> AddSub3/2, Register2/1
  Register3/1 -> AddSub2/2, Register1/1
  AddSub2/1 -> AddSub3/1
  AddSub3/1 -> AddSub6/1
  Register6/1 -> AddSub5/2, Register3/1
  Register5/1 -> AddSub4/2, Register6/1
  Register4/1 -> AddSub1/2, Register5/1
  AddSub1/1 -> AddSub4/1
  AddSub4/1 -> AddSub5/1
  In1/1 -> Register4/1, AddSub1/1
  AddSub9/1 -> Out1/1

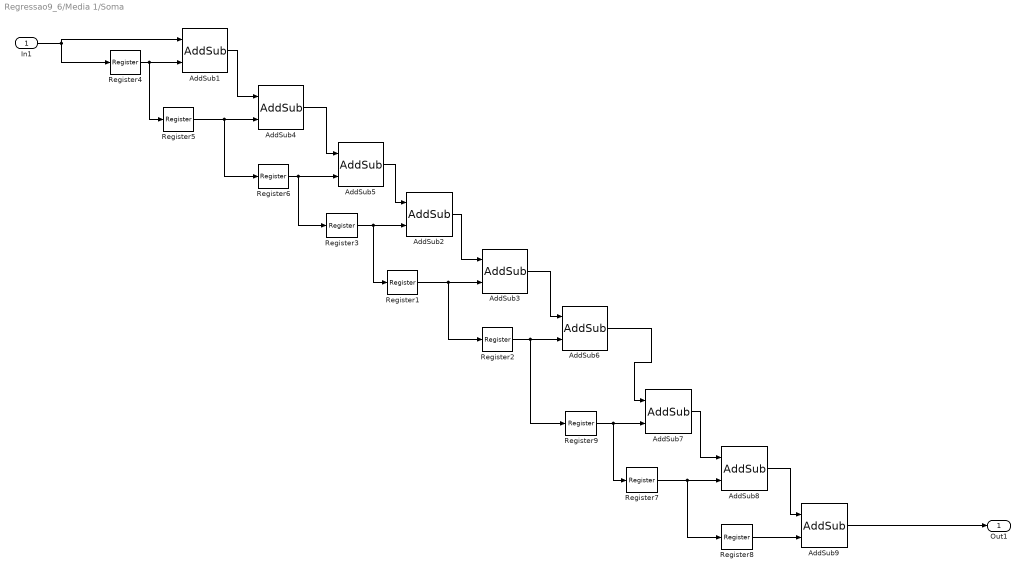
== system Regressao9_6/Media 1/Soma ==
  In1 : Inport
  AddSub{1..9} (9 alike) : xbsIndex_r4/AddSub  mode=Addition  use_carryin=off  use_carryout=off  en=off  latency=0  precision=Full  arith_type=Unsigned  n_bits=16  bin_pt=14  quantization=Truncate  overflow=Wrap  dbl_ovrd=off  use_behavioral_HDL=off  hw_selection=Fabric  pipelined=off  block_type=addsub
  Register{1..9} (9 alike) : xbsIndex_r4/Register  init=0  rst=off  en=off  dbl_ovrd=off  block_type=register
  Out1 : Outport
  wires:
  AddSub9/1 -> Out1/1
  In1/1 -> AddSub1/1, Register4/1
  AddSub4/1 -> AddSub5/1
  AddSub1/1 -> AddSub4/1
  Register4/1 -> Register5/1, AddSub1/2
  Register5/1 -> Register6/1, AddSub4/2
  Register6/1 -> Register3/1, AddSub5/2
  AddSub3/1 -> AddSub6/1
  AddSub2/1 -> AddSub3/1
  Register3/1 -> Register1/1, AddSub2/2
  Register1/1 -> Register2/1, AddSub3/2
  AddSub5/1 -> AddSub2/1
  Register2/1 -> Register9/1, AddSub6/2
  AddSub8/1 -> AddSub9/1
  AddSub7/1 -> AddSub8/1
  Register9/1 -> AddSub7/2, Register7/1
  Register7/1 -> AddSub8/2, Register8/1
  Register8/1 -> AddSub9/2
  AddSub6/1 -> AddSub7/1

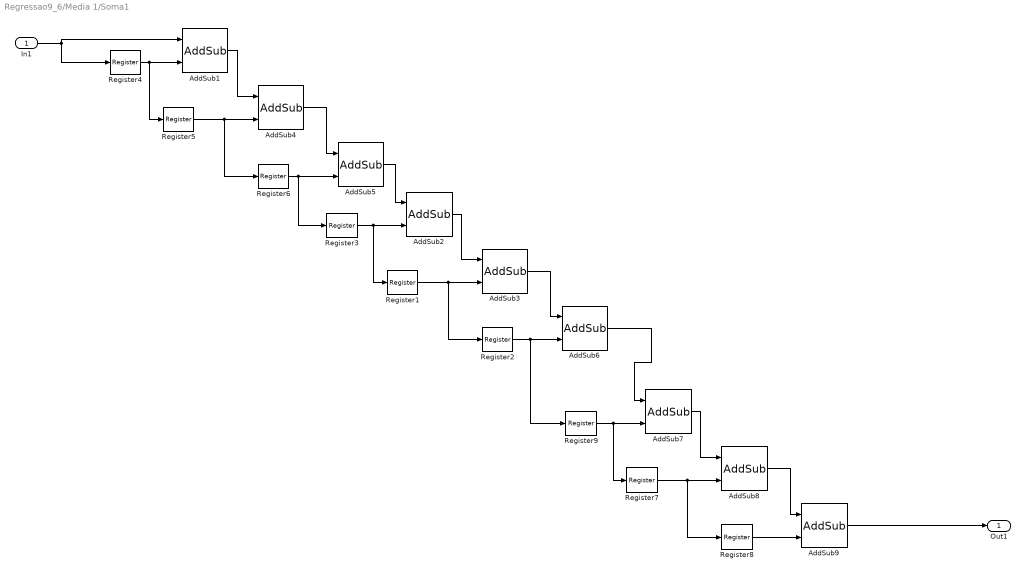
== system Regressao9_6/Media 1/Soma1 ==
  In1 : Inport
  AddSub{1..9} (9 alike) : xbsIndex_r4/AddSub  mode=Addition  use_carryin=off  use_carryout=off  en=off  latency=0  precision=Full  arith_type=Unsigned  n_bits=16  bin_pt=14  quantization=Truncate  overflow=Wrap  dbl_ovrd=off  use_behavioral_HDL=off  hw_selection=Fabric  pipelined=off  block_type=addsub
  Register{1..9} (9 alike) : xbsIndex_r4/Register  init=0  rst=off  en=off  dbl_ovrd=off  block_type=register
  Out1 : Outport
  wires:
  AddSub6/1 -> AddSub7/1
  Register8/1 -> AddSub9/2
  Register7/1 -> Register8/1, AddSub8/2
  Register9/1 -> Register7/1, AddSub7/2
  AddSub7/1 -> AddSub8/1
  AddSub8/1 -> AddSub9/1
  Register2/1 -> AddSub6/2, Register9/1
  AddSub5/1 -> AddSub2/1
  Register1/1 -> AddSub3/2, Register2/1
  Register3/1 -> AddSub2/2, Register1/1
  AddSub2/1 -> AddSub3/1
  AddSub3/1 -> AddSub6/1
  Register6/1 -> AddSub5/2, Register3/1
  Register5/1 -> AddSub4/2, Register6/1
  Register4/1 -> AddSub1/2, Register5/1
  AddSub1/1 -> AddSub4/1
  AddSub4/1 -> AddSub5/1
  In1/1 -> Register4/1, AddSub1/1
  AddSub9/1 -> Out1/1

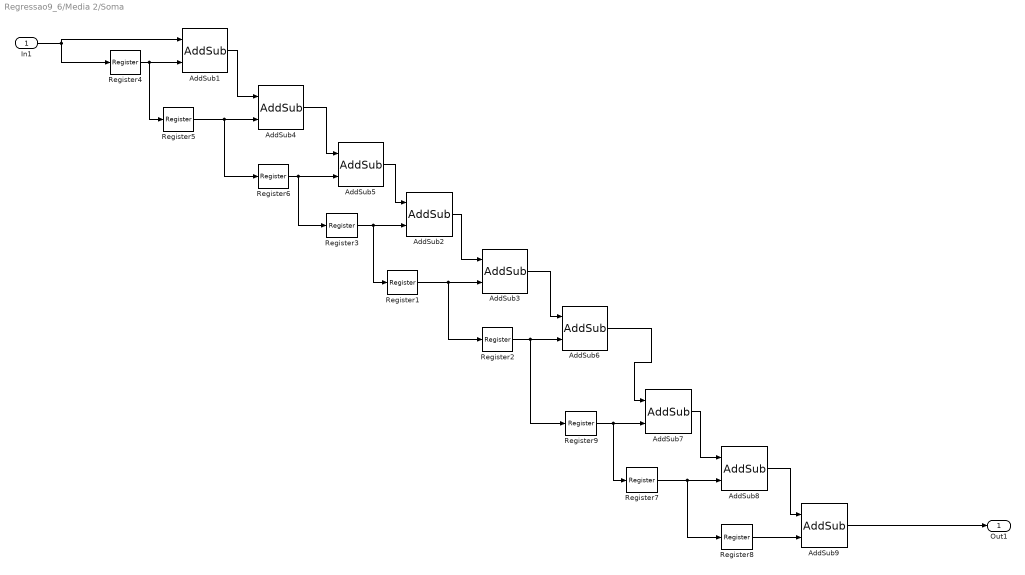
== system Regressao9_6/Media 2/Soma ==
  In1 : Inport
  AddSub{1..9} (9 alike) : xbsIndex_r4/AddSub  mode=Addition  use_carryin=off  use_carryout=off  en=off  latency=0  precision=Full  arith_type=Unsigned  n_bits=16  bin_pt=14  quantization=Truncate  overflow=Wrap  dbl_ovrd=off  use_behavioral_HDL=off  hw_selection=Fabric  pipelined=off  block_type=addsub
  Register{1..9} (9 alike) : xbsIndex_r4/Register  init=0  rst=off  en=off  dbl_ovrd=off  block_type=register
  Out1 : Outport
  wires:
  AddSub9/1 -> Out1/1
  In1/1 -> AddSub1/1, Register4/1
  AddSub4/1 -> AddSub5/1
  AddSub1/1 -> AddSub4/1
  Register4/1 -> Register5/1, AddSub1/2
  Register5/1 -> Register6/1, AddSub4/2
  Register6/1 -> Register3/1, AddSub5/2
  AddSub3/1 -> AddSub6/1
  AddSub2/1 -> AddSub3/1
  Register3/1 -> Register1/1, AddSub2/2
  Register1/1 -> Register2/1, AddSub3/2
  AddSub5/1 -> AddSub2/1
  Register2/1 -> Register9/1, AddSub6/2
  AddSub8/1 -> AddSub9/1
  AddSub7/1 -> AddSub8/1
  Register9/1 -> AddSub7/2, Register7/1
  Register7/1 -> AddSub8/2, Register8/1
  Register8/1 -> AddSub9/2
  AddSub6/1 -> AddSub7/1

== system Regressao9_6/Media 2/Soma1 ==
  In1 : Inport
  AddSub{1..9} (9 alike) : xbsIndex_r4/AddSub  mode=Addition  use_carryin=off  use_carryout=off  en=off  latency=0  precision=Full  arith_type=Unsigned  n_bits=16  bin_pt=14  quantization=Truncate  overflow=Wrap  dbl_ovrd=off  use_behavioral_HDL=off  hw_selection=Fabric  pipelined=off  block_type=addsub
  Register{1..9} (9 alike) : xbsIndex_r4/Register  init=0  rst=off  en=off  dbl_ovrd=off  block_type=register
  Out1 : Outport
  wires:
  AddSub6/1 -> AddSub7/1
  Register8/1 -> AddSub9/2
  Register7/1 -> Register8/1, AddSub8/2
  Register9/1 -> Register7/1, AddSub7/2
  AddSub7/1 -> AddSub8/1
  AddSub8/1 -> AddSub9/1
  Register2/1 -> AddSub6/2, Register9/1
  AddSub5/1 -> AddSub2/1
  Register1/1 -> AddSub3/2, Register2/1
  Register3/1 -> AddSub2/2, Register1/1
  AddSub2/1 -> AddSub3/1
  AddSub3/1 -> AddSub6/1
  Register6/1 -> AddSub5/2, Register3/1
  Register5/1 -> AddSub4/2, Register6/1
  Register4/1 -> AddSub1/2, Register5/1
  AddSub1/1 -> AddSub4/1
  AddSub4/1 -> AddSub5/1
  In1/1 -> Register4/1, AddSub1/1
  AddSub9/1 -> Out1/1

== system Regressao9_6/Media 3/Soma ==
  In1 : Inport
  AddSub{1..9} (9 alike) : xbsIndex_r4/AddSub  mode=Addition  use_carryin=off  use_carryout=off  en=off  latency=0  precision=Full  arith_type=Unsigned  n_bits=16  bin_pt=14  quantization=Truncate  overflow=Wrap  dbl_ovrd=off  use_behavioral_HDL=off  hw_selection=Fabric  pipelined=off  block_type=addsub
  Register{1..9} (9 alike) : xbsIndex_r4/Register  init=0  rst=off  en=off  dbl_ovrd=off  block_type=register
  Out1 : Outport
  wires:
  AddSub9/1 -> Out1/1
  In1/1 -> AddSub1/1, Register4/1
  AddSub4/1 -> AddSub5/1
  AddSub1/1 -> AddSub4/1
  Register4/1 -> Register5/1, AddSub1/2
  Register5/1 -> Register6/1, AddSub4/2
  Register6/1 -> Register3/1, AddSub5/2
  AddSub3/1 -> AddSub6/1
  AddSub2/1 -> AddSub3/1
  Register3/1 -> Register1/1, AddSub2/2
  Register1/1 -> Register2/1, AddSub3/2
  AddSub5/1 -> AddSub2/1
  Register2/1 -> Register9/1, AddSub6/2
  AddSub8/1 -> AddSub9/1
  AddSub7/1 -> AddSub8/1
  Register9/1 -> AddSub7/2, Register7/1
  Register7/1 -> AddSub8/2, Register8/1
  Register8/1 -> AddSub9/2
  AddSub6/1 -> AddSub7/1

== system Regressao9_6/Media 3/Soma1 ==
  In1 : Inport
  AddSub{1..9} (9 alike) : xbsIndex_r4/AddSub  mode=Addition  use_carryin=off  use_carryout=off  en=off  latency=0  precision=Full  arith_type=Unsigned  n_bits=16  bin_pt=14  quantization=Truncate  overflow=Wrap  dbl_ovrd=off  use_behavioral_HDL=off  hw_selection=Fabric  pipelined=off  block_type=addsub
  Register{1..9} (9 alike) : xbsIndex_r4/Register  init=0  rst=off  en=off  dbl_ovrd=off  block_type=register
  Out1 : Outport
  wires:
  AddSub6/1 -> AddSub7/1
  Register8/1 -> AddSub9/2
  Register7/1 -> Register8/1, AddSub8/2
  Register9/1 -> Register7/1, AddSub7/2
  AddSub7/1 -> AddSub8/1
  AddSub8/1 -> AddSub9/1
  Register2/1 -> AddSub6/2, Register9/1
  AddSub5/1 -> AddSub2/1
  Register1/1 -> AddSub3/2, Register2/1
  Register3/1 -> AddSub2/2, Register1/1
  AddSub2/1 -> AddSub3/1
  AddSub3/1 -> AddSub6/1
  Register6/1 -> AddSub5/2, Register3/1
  Register5/1 -> AddSub4/2, Register6/1
  Register4/1 -> AddSub1/2, Register5/1
  AddSub1/1 -> AddSub4/1
  AddSub4/1 -> AddSub5/1
  In1/1 -> Register4/1, AddSub1/1
  AddSub9/1 -> Out1/1

== system Regressao9_6/Media 4/Soma ==
  In1 : Inport
  AddSub{1..9} (9 alike) : xbsIndex_r4/AddSub  mode=Addition  use_carryin=off  use_carryout=off  en=off  latency=0  precision=Full  arith_type=Unsigned  n_bits=16  bin_pt=14  quantization=Truncate  overflow=Wrap  dbl_ovrd=off  use_behavioral_HDL=off  hw_selection=Fabric  pipelined=off  block_type=addsub
  Register{1..9} (9 alike) : xbsIndex_r4/Register  init=0  rst=off  en=off  dbl_ovrd=off  block_type=register
  Out1 : Outport
  wires:
  AddSub9/1 -> Out1/1
  In1/1 -> AddSub1/1, Register4/1
  AddSub4/1 -> AddSub5/1
  AddSub1/1 -> AddSub4/1
  Register4/1 -> Register5/1, AddSub1/2
  Register5/1 -> Register6/1, AddSub4/2
  Register6/1 -> Register3/1, AddSub5/2
  AddSub3/1 -> AddSub6/1
  AddSub2/1 -> AddSub3/1
  Register3/1 -> Register1/1, AddSub2/2
  Register1/1 -> Register2/1, AddSub3/2
  AddSub5/1 -> AddSub2/1
  Register2/1 -> Register9/1, AddSub6/2
  AddSub8/1 -> AddSub9/1
  AddSub7/1 -> AddSub8/1
  Register9/1 -> AddSub7/2, Register7/1
  Register7/1 -> AddSub8/2, Register8/1
  Register8/1 -> AddSub9/2
  AddSub6/1 -> AddSub7/1

== system Regressao9_6/Media 4/Soma1 ==
  In1 : Inport
  AddSub{1..9} (9 alike) : xbsIndex_r4/AddSub  mode=Addition  use_carryin=off  use_carryout=off  en=off  latency=0  precision=Full  arith_type=Unsigned  n_bits=16  bin_pt=14  quantization=Truncate  overflow=Wrap  dbl_ovrd=off  use_behavioral_HDL=off  hw_selection=Fabric  pipelined=off  block_type=addsub
  Register{1..9} (9 alike) : xbsIndex_r4/Register  init=0  rst=off  en=off  dbl_ovrd=off  block_type=register
  Out1 : Outport
  wires:
  AddSub6/1 -> AddSub7/1
  Register8/1 -> AddSub9/2
  Register7/1 -> Register8/1, AddSub8/2
  Register9/1 -> Register7/1, AddSub7/2
  AddSub7/1 -> AddSub8/1
  AddSub8/1 -> AddSub9/1
  Register2/1 -> AddSub6/2, Register9/1
  AddSub5/1 -> AddSub2/1
  Register1/1 -> AddSub3/2, Register2/1
  Register3/1 -> AddSub2/2, Register1/1
  AddSub2/1 -> AddSub3/1
  AddSub3/1 -> AddSub6/1
  Register6/1 -> AddSub5/2, Register3/1
  Register5/1 -> AddSub4/2, Register6/1
  Register4/1 -> AddSub1/2, Register5/1
  AddSub1/1 -> AddSub4/1
  AddSub4/1 -> AddSub5/1
  In1/1 -> Register4/1, AddSub1/1
  AddSub9/1 -> Out1/1

== system Regressao9_6/Media 5/Soma ==
  In1 : Inport
  AddSub{1..9} (9 alike) : xbsIndex_r4/AddSub  mode=Addition  use_carryin=off  use_carryout=off  en=off  latency=0  precision=Full  arith_type=Unsigned  n_bits=16  bin_pt=14  quantization=Truncate  overflow=Wrap  dbl_ovrd=off  use_behavioral_HDL=off  hw_selection=Fabric  pipelined=off  block_type=addsub
  Register{1..9} (9 alike) : xbsIndex_r4/Register  init=0  rst=off  en=off  dbl_ovrd=off  block_type=register
  Out1 : Outport
  wires:
  AddSub9/1 -> Out1/1
  In1/1 -> AddSub1/1, Register4/1
  AddSub4/1 -> AddSub5/1
  AddSub1/1 -> AddSub4/1
  Register4/1 -> Register5/1, AddSub1/2
  Register5/1 -> Register6/1, AddSub4/2
  Register6/1 -> Register3/1, AddSub5/2
  AddSub3/1 -> AddSub6/1
  AddSub2/1 -> AddSub3/1
  Register3/1 -> Register1/1, AddSub2/2
  Register1/1 -> Register2/1, AddSub3/2
  AddSub5/1 -> AddSub2/1
  Register2/1 -> Register9/1, AddSub6/2
  AddSub8/1 -> AddSub9/1
  AddSub7/1 -> AddSub8/1
  Register9/1 -> AddSub7/2, Register7/1
  Register7/1 -> AddSub8/2, Register8/1
  Register8/1 -> AddSub9/2
  AddSub6/1 -> AddSub7/1

== system Regressao9_6/Media 5/Soma1 ==
  In1 : Inport
  AddSub{1..9} (9 alike) : xbsIndex_r4/AddSub  mode=Addition  use_carryin=off  use_carryout=off  en=off  latency=0  precision=Full  arith_type=Unsigned  n_bits=16  bin_pt=14  quantization=Truncate  overflow=Wrap  dbl_ovrd=off  use_behavioral_HDL=off  hw_selection=Fabric  pipelined=off  block_type=addsub
  Register{1..9} (9 alike) : xbsIndex_r4/Register  init=0  rst=off  en=off  dbl_ovrd=off  block_type=register
  Out1 : Outport
  wires:
  AddSub6/1 -> AddSub7/1
  Register8/1 -> AddSub9/2
  Register7/1 -> Register8/1, AddSub8/2
  Register9/1 -> Register7/1, AddSub7/2
  AddSub7/1 -> AddSub8/1
  AddSub8/1 -> AddSub9/1
  Register2/1 -> AddSub6/2, Register9/1
  AddSub5/1 -> AddSub2/1
  Register1/1 -> AddSub3/2, Register2/1
  Register3/1 -> AddSub2/2, Register1/1
  AddSub2/1 -> AddSub3/1
  AddSub3/1 -> AddSub6/1
  Register6/1 -> AddSub5/2, Register3/1
  Register5/1 -> AddSub4/2, Register6/1
  Register4/1 -> AddSub1/2, Register5/1
  AddSub1/1 -> AddSub4/1
  AddSub4/1 -> AddSub5/1
  In1/1 -> Register4/1, AddSub1/1
  AddSub9/1 -> Out1/1
